simulink model "qpsk_modulation_and_demodulation"  (R2024a)
settings: Solver=VariableStepAuto  StartTime=0.0  StopTime=0.0001  RelTol=1e-3
libraries: commrfcorlib x2, dspfdesign x2, commrflib2 x2, commdigbbndpm3 x2, commfilt2 x2, dspsigops x2, commchan3 x1, commrandsrc3 x1, simulink x1, commsync2 x1, whdlio x1
settings Model: Creator=digital  LastModifiedBy=digital

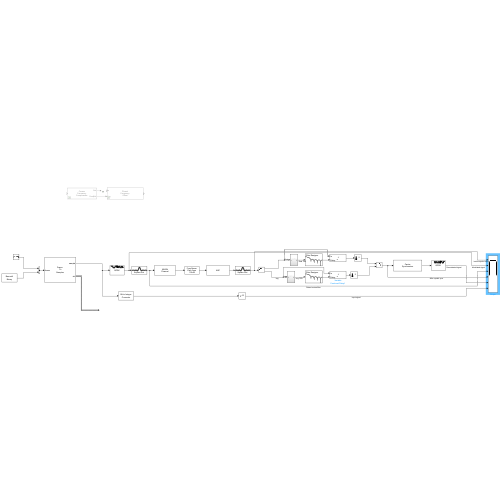
[thumbnail: Simulink's stored preview of the top-level diagram]
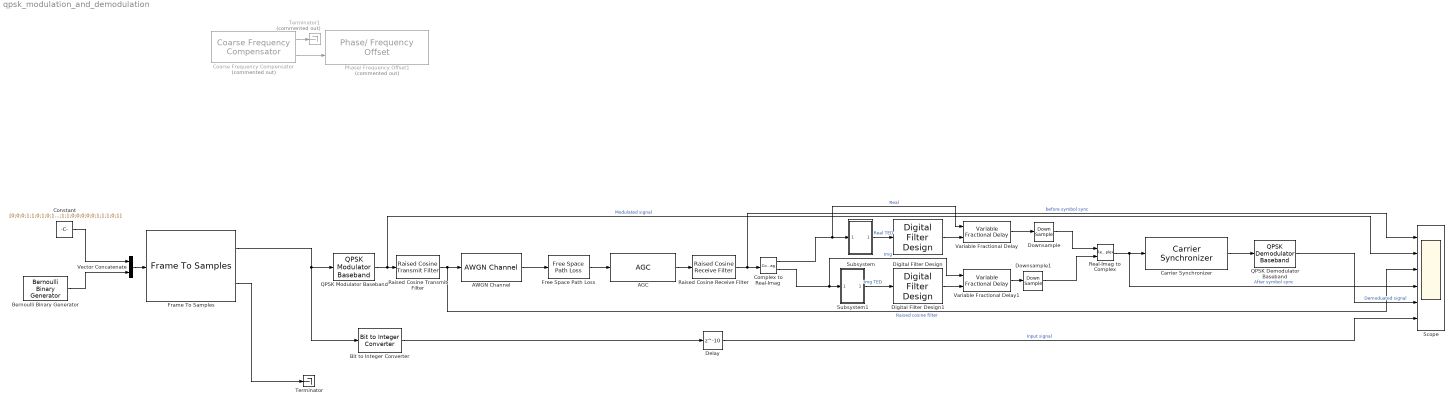
== system qpsk_modulation_and_demodulation ==
  AGC : commrfcorlib/AGC  LegacyMode=off  DetectorMethod=Rectifier  LoopMethod=Linear  UpdatePeriod=100  StepSize=0.1  AdaptationStepSize=0.01  DesiredOutputPower=1  AveragingLength=100  MaximumGain=30  MaxPowerGain=60  GainOutputPort=off  InputPowerOutputPort=off  SimulateUsing=Interpreted execution
  AWGN Channel : commchan3/AWGN Channel  LegacyMode=off  NoiseMethod="Signal to noise ratio  (SNR)"  noiseMode="Signal to noise ratio  (SNR)"  EbNo=10  EsNo=10  SNR=15  BitsPerSymbol=1  SignalPower=1  SamplesPerSymbol=1  SymbolPeriod=1  VarianceSource=Parameter  Variance=1  RandomStream=Global stream  Seed=67  SimulateUsing=Interpreted execution
  Bernoulli Binary Generator : commrandsrc3/Bernoulli Binary Generator  ProbabilityOfZero=0.5  SeedSource=Auto  Seed=0  SampleTime=128/10e6  SamplesPerFrame=96  OutputDataType=double  SimulateUsing=Interpreted execution
  Bit to Integer Converter : simulink/Logic and Bit Operations/Bit to Integer Converter  nbits=2  bitOrder=MSB first  signedOutputValues=Unsigned  outDtype=Inherit via internal rule  outDtypeSigned=Inherit via internal rule
  Carrier Synchronizer : commsync2/Carrier Synchronizer  Modulation=QPSK  ModulationPhaseOffset=Auto  CustomPhaseOffset=0  SamplesPerSymbol=2  DampingFactor=0.707  NormalizedLoopBandwidth=0.01  EstimatedPhaseErrorOutputPort=off  SimulateUsing=Interpreted execution
  Coarse Frequency Compensator : commrfcorlib/Coarse Frequency Compensator  Commented=on  Modulation=QPSK  Algorithm=FFT-based  FrequencyResolution=100  MaximumFrequencyOffset=5e3  SamplesPerSymbol=4  EstimatedFreqOffsetPort=on  SimulateUsing=Interpreted execution
      settings: LibrarySourceBlock=|
      | commsync2/Coarse Frequency
      | Compensator
  Complex to Real-Imag : ComplexToRealImag
  Constant : Constant  Value=[0;0;0;1;1;0;1;0;1;1;0;0;1;1;1;1;1;1;1;1;1;1;0;0;0;0;0;1;1;1;0;1]  OutDataTypeStr=double  SampleTime=128/10e6
  Delay : Delay  DelayLength=10  InitialCondition=0
  Digital Filter Design : dspfdesign/Digital Filter Design  mwdsp_browser_bugfix_var=off
  Digital Filter Design1 : dspfdesign/Digital Filter Design  mwdsp_browser_bugfix_var=off
  Downsample : DownSample  AllowArbitraryFixedInput=on
  Downsample1 : DownSample  AllowArbitraryFixedInput=on
  Frame To Samples : whdlio/Frame To Samples  InterSampleIdleCycles=0  InterFrameIdleCycles=0  OutputSize=2  InterleaveSamples=off
  Free Space Path Loss : commrflib2/Free Space Path Loss  mode=Distance and Frequency  dB=10  d=10  fc=1920
  Phase/ Frequency Offset1 : commrflib2/Phase// Frequency Offset  Commented=on  phaseOffset=0  freqPort=on  freqOffset=0
      settings: LibrarySourceBlock=|
      | commrfcorlib/Phase//
      | Frequency
      | Offset
  QPSK Demodulator Baseband : commdigbbndpm3/QPSK Demodulator Baseband  OutType=Integer  DecType=Hard decision  VarSource=Dialog  Variance=1  Dec=Gray  Ph=pi/4  outDtype1=Inherit via internal rule  outDtype2=Inherit via internal rule  derotateFactorWordLen=16  derotateFactorDataTypeStr=Inherit: Same word length as input  derotateFactorLastDataTypeStr=Inherit: Same word length as input
  QPSK Modulator Baseband : commdigbbndpm3/QPSK Modulator Baseband  InType=Bit  Enc=Gray  Ph=pi/4  outDtype=double  outWordLen=16  outUDDataType=sfix(16)  outFracLenMode=Best precision  outFracLen=15  outDataTypeStr=double  outLastDataTypeStr=double
  Raised Cosine Receive Filter : commfilt2/Raised Cosine Receive Filter  filtType=Square root  R=0.2  filtSpan=10  N=16  downFactor=8  downOffset=0  filterGain=1  RateOptions=Allow multirate processing  framing=Mute  checkCoeff=off  variableName=rcRxFilt  currentFiltSpan=10  D=5  inputOffset=0  sampMode=Mute  saveAsFlag=0  rateMode=Downsampling  checkGain=Normalized  launchFVT=on  roundingMode=Floor  overflowMode=off  coeffDataTypeStr=Inherit: Same word length as input  coeffMin=[]  coeffMax=[]  coeffLastDataTypeStr=Inherit: Same word length as input  accumDataTypeStr=Inherit: Same as product output  accumLastDataTypeStr=Inherit: Same as product output  outputDataTypeStr=Inherit: Same as accumulator  outputMin=[]  outputMax=[]  outputLastDataTypeStr=Inherit: Same as accumulator
  Raised Cosine Transmit Filter : commfilt2/Raised Cosine Transmit Filter  filtType=Square root  R=0.2  filtSpan=10  N=16  filterGain=1  RateOptions=Allow multirate processing  framing=Mute  checkCoeff=off  variableName=rcTxFilt  checkGain=Normalized  sampMode=Mute  saveAsFlag=0  currentFiltSpan=10  D=(10)/2  launchFVT=on  roundingMode=Floor  overflowMode=off  coeffDataTypeStr=Inherit: Same word length as input  coeffMin=[]  coeffMax=[]  coeffLastDataTypeStr=Inherit: Same word length as input  outputDataTypeStr=Inherit: Same as accumulator  outputMin=[]  outputMax=[]  outputLastDataTypeStr=Inherit: Same as accumulator
  Real-Imag to Complex : RealImagToComplex
  Scope : Scope  NumInputPorts=6
  Subsystem : Subsystem
  Subsystem1 : Subsystem
  Terminator : Terminator
  Terminator1 : Terminator  Commented=on
  Variable Fractional Delay : dspsigops/Variable Fractional Delay  mode=OBSOLETE  modeActive=Linear  L=4  FarrowL=4  R=10  alpha=1  dmax=100  ic=0  noDFT=off  fallbackFIR=Clip to the minimum value necessary for centered kernel  fallbackFarrow=Clip to the minimum value necessary for centered kernel  roundingMode=Zero  overflowMode=off
  Variable Fractional Delay1 : dspsigops/Variable Fractional Delay  mode=OBSOLETE  modeActive=Linear  L=4  FarrowL=4  R=10  alpha=1  dmax=100  ic=0  noDFT=off  fallbackFIR=Clip to the minimum value necessary for centered kernel  fallbackFarrow=Clip to the minimum value necessary for centered kernel  roundingMode=Zero  overflowMode=off
  Vector Concatenate : Concatenate
  wires:
  Constant/1 -> Vector Concatenate/1
  Bernoulli Binary Generator/1 -> Vector Concatenate/2
  Frame To Samples/1 -> Bit to Integer Converter/1, QPSK Modulator Baseband/1
  Raised Cosine Transmit Filter/1 -> Scope/3, AWGN Channel/1  "Raised cosine filter"
  AWGN Channel/1 -> Free Space Path Loss/1
  Free Space Path Loss/1 -> AGC/1
  Frame To Samples/2 -> Terminator/1
  Vector Concatenate/1 -> Frame To Samples/1
  AGC/1 -> Raised Cosine Receive Filter/1
  Bit to Integer Converter/1 -> Delay/1
  Coarse Frequency Compensator/2 -> Phase/ Frequency Offset1/2
  Coarse Frequency Compensator/1 -> Terminator1/1
  Delay/1 -> Scope/6  "Input signal"
  Raised Cosine Receive Filter/1 -> Scope/1, Complex to Real-Imag/1  "before symbol sync"
  Complex to Real-Imag/1 -> Variable Fractional Delay/1, Subsystem/1(In1)  "Real"
  Complex to Real-Imag/2 -> Variable Fractional Delay1/1, Subsystem1/1(In1)  "Img"
  Subsystem1/1(Out1) -> Digital Filter Design1/1  "Img TED"
  Subsystem/1(Out1) -> Digital Filter Design/1  "Real TED"
  Digital Filter Design/1 -> Variable Fractional Delay/2
  Digital Filter Design1/1 -> Variable Fractional Delay1/2
  Variable Fractional Delay1/1 -> Downsample1/1
  Variable Fractional Delay/1 -> Downsample/1
  Downsample/1 -> Real-Imag to Complex/1
  Real-Imag to Complex/1 -> Scope/4, Carrier Synchronizer/1  "After symbol sync"
  Downsample1/1 -> Real-Imag to Complex/2
  Carrier Synchronizer/1 -> QPSK Demodulator Baseband/1
  QPSK Demodulator Baseband/1 -> Scope/5  "Demoduated signal"
  QPSK Modulator Baseband/1 -> Scope/2, Raised Cosine Transmit Filter/1  "Modulated signal"

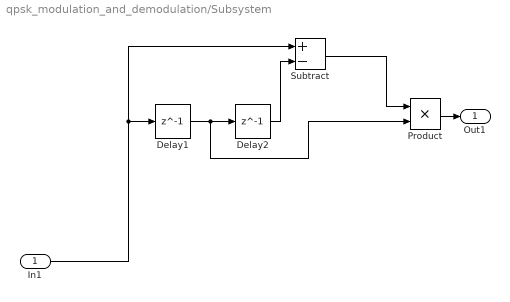
== system qpsk_modulation_and_demodulation/Subsystem ==
  In1 : Inport
  Delay1 : Delay  DelayLength=1  InitialCondition=0
  Delay2 : Delay  DelayLength=1  InitialCondition=0
  Product : Product
  Subtract : Sum  Inputs=+-
  Out1 : Outport
  wires:
  Product/1 -> Out1/1
  Delay1/1 -> Product/2, Delay2/1
  In1/1 -> Subtract/1, Delay1/1
  Subtract/1 -> Product/1
  Delay2/1 -> Subtract/2

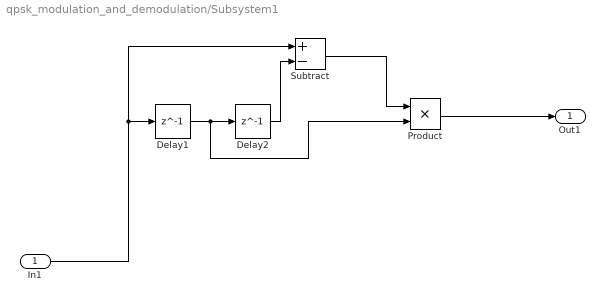
== system qpsk_modulation_and_demodulation/Subsystem1 ==
  In1 : Inport
  Delay1 : Delay  DelayLength=1  InitialCondition=0
  Delay2 : Delay  DelayLength=1  InitialCondition=0
  Product : Product
  Subtract : Sum  Inputs=+-
  Out1 : Outport
  wires:
  Delay2/1 -> Subtract/2
  Subtract/1 -> Product/1
  In1/1 -> Delay1/1, Subtract/1
  Delay1/1 -> Delay2/1, Product/2
  Product/1 -> Out1/1
